simulink model "interpolation_nD_TestGen14"  (R2017b)
settings: Solver=FixedStepDiscrete  StartTime=0.0  StopTime=10.0  RelTol=1e-3
PreLoadFcn:
  |  LUTObj = Simulink.LookupTable;
  |  LUTObj.Table.Value = [35.6168797288049;52.2613294330982;108.402364211025];
  |  LUTObj.Table.DataType = 'auto';
  |  LUTObj.StructTypeInfo.Name = 'myLUTStruct';
  |  LUTObj.BreakpointsSpecification = 'Reference';
  |  LUTObj.Breakpoints{1} = 'myBpSet1';
  | myBpSet1 = Simulink.Breakpoint;
  | myBpSet1.Breakpoints.Value = [1 2 3];
undefined symbols (not defined in the file): Block_TestLib, reset
settings Model: Creator=ktrinh  LastModifiedBy=ktrinh
settings DebuggingCC: ParameterOverflowMsg=none

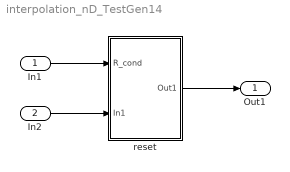
== system interpolation_nD_TestGen14 ==
  In1 : Inport
  In2 : Inport  Port=2  OutDataTypeStr=Bus: kfBus  BusOutputAsStruct=on
  reset : Subsystem  AncestorBlock=Block_TestLib/reset
  Out1 : Outport
  wires:
  In1/1 -> reset/1(R_cond)
  In2/1 -> reset/2(In1)
  reset/1(Out1) -> Out1/1

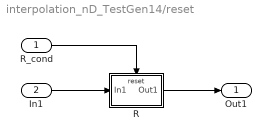
== system interpolation_nD_TestGen14/reset ==
  R_cond : Inport  OutDataTypeStr=boolean
  In1 : Inport  Port=2  OutDataTypeStr=Bus: kfBus  BusOutputAsStruct=on
  R : Subsystem  TreatAsAtomicUnit=on
  Out1 : Outport
  wires:
  R_cond/1 -> R/Reset
  In1/1 -> R/1(In1)
  R/1(Out1) -> Out1/1

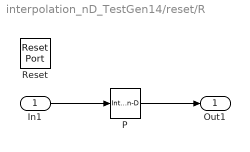
== system interpolation_nD_TestGen14/reset/R ==
  In1 : Inport  OutMin=0  OutMax=3  OutDataTypeStr=Bus: kfBus  PortDimensions=1  BusOutputAsStruct=on
  Reset : ResetPort  DisableCoverage=on
  P : Interpolation_n-D  InitFcn=|  NumberOfTableDimensions=1  Table=[35.6168797288049;52.2613294330982;108.402364211025]  TableSpecification=Lookup table object  LookupTableObject=LUTObj  InterpMethod=Flat  RequireIndexFractionAsBus=on  OutDataTypeStr=int8  InternalRulePriority=Speed  RndMeth=Ceiling  IntermediateResultsDataTypeStr=int32
      | elems(1) = Simulink.BusElement;
      | elems(1).Name = 'Index';
      | elems(1).DataType = 'int8';
      | elems(2) = Simulink.BusElement;
      | elems(2).Name = 'Fraction';
      | elems(2).DataType = 'double';
      | kfBus = Simulink.Bus;
      | kfBus.Elements = elems;
      | clear elems;
      | assignin('base', 'kfBus', kfBus);
      settings: InputPortMap=u0
  Out1 : Outport
  wires:
  In1/1 -> P/1
  P/1 -> Out1/1
